simulink model "wrench_observer_R2016b"  (R2016b)
settings: Solver=VariableStepAuto  StartTime=0.0  StopTime=0.75  RelTol=1e-3
InitFcn:
  | %x_k1 = 0.00001*ones(36,1); % initialisation with initial state uncertainity
  | %P_k1 = 0.00001*ones(36); % initialisation with initial state uncertainity
values from neighbouring files (symbols this model uses):
  a_noise = 0    [parameter.m]
  alpha1 = pi/2    (= 1.57079632679)    [parameter.m]
  alpha2 = 0    [parameter.m]
  alpha3 = 0    [parameter.m]
  angular_noise = 0    [parameter.m]
  g = 9.81    [parameter.m]
  K_f_comm = 1    [parameter.m]
  K_I = [500*eye(3), zeros(3), zeros(3) ... (first row only)    [parameter.m]
  K_tau_comm = 1    [parameter.m]
  K_tau_man_comm = 1    [parameter.m]
  m = 3.9    [parameter.m]
  m_l1 = 0.3    [parameter.m]
  m_l2 = 0.35    [parameter.m]
  m_l3 = 0.35    [parameter.m]
  N_m = 1*diag([(p_noise/(3*noise_factor))^2 (p_noise/(3*noise_factor))^2 (p_noise/(3*noise_factor))^2 (a_noise/(3*noise_factor))^2 (a_noise/(3*noise_factor))^2 (a_noise/(3*noise_factor))^2 (angular_noise/(3*noise_factor))^2 (angular_noise/(3*noise_factor))^2 (angular_noise/(3*noise_factor))^2 (omega_noise/(3*noise_factor))^2 (omega_noise/(3*noise_factor))^2 (omega_noise/(3*noise_factor))^2 (theta_noise/( ...(+272 chars)    [parameter.m]
  N_p = diag(noise_factor_EKF)    [parameter.m]
  omega_dot_noise = 0    [parameter.m]
  omega_noise = 0    [parameter.m]
  p_L1_l1 = [p_L1_x_l1 p_L1_y_l1 p_L1_z_l1]'    [parameter.m]
  p_L2_l2 = [p_L2_x_l2 p_L2_y_l2 p_L2_z_l2]'    [parameter.m]
  p_L3_l3 = [p_L3_x_l3 p_L3_y_l3 p_L3_z_l3]'    [parameter.m]
  p_noise = 0    [parameter.m]
  R_B_L0 = [1 0 0;0 1 0; 0 0 1]    [parameter.m]
  T_delay = 0    [parameter.m]
  T_dis = 0.01    [parameter.m]
  theta_dot_dot_noise = 0    [parameter.m]
  theta_dot_noise = 0    [parameter.m]
  theta_noise = 0    [parameter.m]
  Ts = 1/250    (= 0.004)    [parameter.m]
  v_noise = 0    [parameter.m]
libraries: simulink x9, dspstat3 x2, dspinverses x1
(part 3 of 5)

== matlab function wrench_observer_R2016b/Wrench Observer EKF/MATLAB Function1 ==
  data: T_dis input; F output
function F = fcn(T_dis)
F = [ 	1, 	0, 	0, 	T_dis, 	0, 	0, 	0, 	0, 	0, 	0, 	0, 	0, 	0, 	0, 	0, 	0, 	0, 	0, 	0, 	0, 	0, 	0, 	0, 	0, 	0, 	0, 	0, 	0, 	0, 	0, 	0, 	0, 	0, 	0, 	0, 	0; 
		0, 	1, 	0, 	0, 	T_dis, 	0, 	0, 	0, 	0, 	0, 	0, 	0, 	0, 	0, 	0, 	0, 	0, 	0, 	0, 	0, 	0, 	0, 	0, 	0, 	0, 	0, 	0, 	0, 	0, 	0, 	0, 	0, 	0, 	0, 	0, 	0; 
		0, 	0, 	1, 	0, 	0, 	T_dis, 	0, 	0, 	0, 	0, 	0, 	0, 	0, 	0, 	0, 	0, 	0, 	0, 	0, 	0, 	0, 	0, 	0, 	0, 	0, 	0, 	0, 	0, 	0, 	0, 	0, 	0, 	0, 	0, 	0, 	0; 
		0, 	0, 	0, 	1, 	0, 	0, 	-(10*T_dis*((21*3^(1/2))/10000000000 + (3^(1/2)*((3*3^(1/2))/20 - 1/10))/2000000 - 3783/80000000000))/49, 	-(10*T_dis*((63*3^(1/2))/40000000000 + (3^(1/2)*((3*3^(1/2))/20 - 1/10))/2000000 + 52641/160000000000))/49, 	-(10*T_dis*((21*3^(1/2))/40000000000 + (3^(1/2)*((3*3^(1/2))/20 - 1/10))/1000000 + 53013/160000000000))/49, 	-(10*T_dis*((21*3^(1/2))/4000000 + 3/2000000))/49, 	(381*T_dis)/7840000, 	-(10*T_dis*((21*3^(1/2))/4000000 + (3^(1/2)*((3*3^(1/2))/20 - 1/10))/400 + 237/32000000))/49, 	(10*T_dis*((35937*3^(1/2))/1600000000000 + 1/100000000))/49, 	(10*T_dis*((35397*3^(1/2))/1600000000000 + 63/40000000000))/49, 	(10*T_dis*((177*3^(1/2))/80000000000 + 21/25000000000))/49, 	-(10*T_dis*((3*3^(1/2)*((3*3^(1/2))/20 - 1/10))/400 + 27/40000))/49, 	-(687*T_dis)/1600000, 	-(23643*T_dis)/156800000, 	(10*T_dis)/49, 	0, 	0, 	(10*T_dis)/49, 	0, 	0, 	0, 	0, 	0, 	0, 	0, 	0, 	0, 	0, 	0, 	0, 	0, 	0; 
		0, 	0, 	0, 	0, 	1, 	0, 	-(10*T_dis*((243969*3^(1/2))/800000000000 + 26389/50000000000))/49, 	(10*T_dis*((26073*3^(1/2))/400000000000 - 991/12500000000))/49, 	-(10*T_dis*((179727*3^(1/2))/800000000000 + 110003/200000000000))/49, 	-(381*T_dis)/784000, 	-(10*T_dis*((2121*3^(1/2))/80000000 + 303/40000000))/49, 	(10*T_dis*((56073*3^(1/2))/160000000 - 10303/40000000))/49, 	-(10*T_dis*((3^(1/2)*((3*3^(1/2))/20 - 1/10))/10000000 + 60189/1600000000000))/49, 	(10*T_dis*((249*3^(1/2))/80000000000 - 192873/1600000000000))/49, 	-(10*T_dis*((3561*3^(1/2))/160000000000 + 990219/8000000000000))/49, 	(10*T_dis*((3*3^(1/2))/8000 - 3/2000))/49, 	-(10*T_dis*((35979*3^(1/2))/16000000 + 3/2000))/49, 	-(10*T_dis*((23979*3^(1/2))/32000000 + 21/160000))/49, 	0, 	(10*T_dis)/49, 	0, 	0, 	(10*T_dis)/49, 	0, 	0, 	0, 	0, 	0, 	0, 	0, 	0, 	0, 	0, 	0, 	0, 	0; 
		0, 	0, 	0, 	0, 	0, 	1, 	(10*T_dis*((39969*3^(1/2))/80000000000 + (3^(1/2)*((3*3^(1/2))/20 - 1/10))/2000000 + 5337/40000000000))/49, 	(10*T_dis*((3^(1/2)*((3*3^(1/2))/20 - 1/10))/2000000 - (24273*3^(1/2))/80000000000 + 10003/20000000000))/49, 	(10*T_dis*((3927*3^(1/2))/80000000000 + 5331/40000000000))/49, 	(10*T_dis*((21*3^(1/2))/40000 + (3^(1/2)*((3*3^(1/2))/20 - 1/10))/400 + 237/320000))/49, 	-(10*T_dis*((60231*3^(1/2))/16000000 - 5003/2000000))/49, 	0, 	(10*T_dis*((183*3^(1/2))/16000000000 + (3^(1/2)*((3*3^(1/2))/20 - 1/10))/2000000 - 611/160000000000))/49, 	-(10*T_dis*((14871*3^(1/2))/800000000000 - 24147/160000000000))/49, 	-(10*T_dis*((24021*3^(1/2))/1600000000000 - 17601/200000000000))/49, 	(10*T_dis*((3^(1/2)*((3*3^(1/2))/20 - 1/10))/400 - (9*3^(1/2))/4000 + 1/400))/49, 	(10*T_dis*((2379*3^(1/2))/1600000 + 63/160000))/49, 	(10*T_dis*((4779*3^(1/2))/3200000 + 63/320000))/49, 	0, 	0, 	(10*T_dis)/49, 	0, 	0, 	(10*T_dis)/49, 	0, 	0, 	0, 	0, 	0, 	0, 	0, 	0, 	0, 	0, 	0, 	0; 
		0, 	0, 	0, 	0, 	0, 	0, 	(T_dis*(cos(1/10)/100000 - sin(1/10)/100000))/(cos(1/10)^2 + sin(1/10)^2) + 1, 	0, 	0, 	T_dis, 	(T_dis*sin(1/10))/(cos(1/10)^2 + sin(1/10)^2), 	(T_dis*cos(1/10))/(cos(1/10)^2 + sin(1/10)^2), 	0, 	0, 	0, 	0, 	0, 	0, 	0, 	0, 	0, 	0, 	0, 	0, 	0, 	0, 	0, 	0, 	0, 	0, 	0, 	0, 	0, 	0, 	0, 	0; 
		0, 	0, 	0, 	0, 	0, 	0, 	-(T_dis*(cos(1/10)/100000 + sin(1/10)/100000))/(cos(1/10)^2 + sin(1/10)^2), 	1, 	0, 	0, 	(T_dis*cos(1/10))/(cos(1/10)^2 + sin(1/10)^2), 	-(T_dis*sin(1/10))/(cos(1/10)^2 + sin(1/10)^2), 	0, 	0, 	0, 	0, 	0, 	0, 	0, 	0, 	0, 	0, 	0, 	0, 	0, 	0, 	0, 	0, 	0, 	0, 	0, 	0, 	0, 	0, 	0, 	0; 
		0, 	0, 	0, 	0, 	0, 	0, 	(T_dis*(cos(1/10)/100000 - sin(1/10)/100000))/(cos(1/10)*(cos(1/10)^2 + sin(1/10)^2)), 	(T_dis*sin(1/10)*(cos(1/10)/100000 + sin(1/10)/100000))/(cos(1/10)^2*(cos(1/10)^2 + sin(1/10)^2)), 	1, 	0, 	(T_dis*sin(1/10))/(cos(1/10)*(cos(1/10)^2 + sin(1/10)^2)), 	T_dis/(cos(1/10)^2 + sin(1/10)^2), 	0, 	0, 	0, 	0, 	0, 	0, 	0, 	0, 	0, 	0, 	0, 	0, 	0, 	0, 	0, 	0, 	0, 	0, 	0, 	0, 	0, 	0, 	0, 	0; 
		0, 	0, 	0, 	-T_dis*((5678455*3^(1/2))/877074 - 11415/292358), 	T_dis*((41050000000*3^(1/2)*((2121*3^(1/2))/80000000 + 303/40000000))/1315611 + 32247375/584716), 	T_dis*((41050000000*3^(1/2)*((11937*3^(1/2))/3200000 - 1/400))/1315611 - (9512500*3^(1/2)*((3*3^(1/2))/20 - 1/10))/146179 + 17978625/1169432), 	-T_dis*((41050000000*3^(1/2)*((3185121*3^(1/2))/1600000000000000 + 28784631/800000000000000))/1315611 - (20898335275230313*3^(1/2))/32821708862976000000 + (124478660218750000*3^(1/2)*((1196771067*3^(1/2))/16000000000000000 + 638273444637/32000000000000000))/192314700369 + (24547528595*3^(1/2)*((3*3^(1/2))/20 - 1/10))/4102713607872 + 268511624179821543629/656434177259520000000), 	-T_dis*((63720582757786447*3^(1/2))/98465126588928000000 - (41050000000*3^(1/2)*((1199798391*3^(1/2))/1600000000000000 - 3443358149/6400000000000000))/1315611 + (192991315468750000*3^(1/2)*((1196771067*3^(1/2))/16000000000000000 + 638273444637/32000000000000000))/576944101107 - (79106538965*3^(1/2)*((3*3^(1/2))/20 - 1/10))/12308140823616 + 20428475245687929968893/1969302531778560000000), 	-T_dis*((41050000000*3^(1/2)*((12396063*3^(1/2))/3200000000000000 + 59490177/1280000000000000))/1315611 + (31780980385867259*3^(1/2))/24616281647232000000 + (333669896375000000*3^(1/2)*((1196771067*3^(1/2))/16000000000000000 + 638273444637/32000000000000000))/576944101107 - (38681210545*3^(1/2)*((3*3^(1/2))/20 - 1/10))/3077035205904 + 4954579914681820686731/492325632944640000000), 	1 - (1927715899*3^(1/2)*T_dis)/5613273600, 	(1655290277*T_dis)/18710912000, 	T_dis*((17996889*3^(1/2))/467772800 + (41050000000*3^(1/2)*((16870959*3^(1/2))/640000000000 + 2152887/640000000000))/1315611 + 2040702927/18710912000), 	-T_dis*((278322450041*3^(1/2))/58471600000000 + (41050000000*3^(1/2)*((3^(1/2)*((3*3^(1/2))/20 - 1/10))/4000000 - (395710537*3^(1/2))/16000000000000000 + 3530354301/32000000000000000))/1315611 + (8210000000*3^(1/2)*((3935023*3^(1/2))/1600000000000000 - (3^(1/2)*((3*3^(1/2))/20 - 1/10))/40000000 + 641376324757/32000000000000000))/1315611 + 174654816435461/140331840000000), 	-T_dis*((41050000000*3^(1/2)*((108595719*3^(1/2))/4000000000000000 + 352356880263/1600000000000000000))/1315611 - (98168671543069*3^(1/2))/50659312000000000 + (2800*3^(1/2)*((3*3^(1/2))/20 - 1/10))/3166207 + 34794801151665391/49139532640000000), 	-T_dis*((41050000000*3^(1/2)*((498635583*3^(1/2))/32000000000000000 + 473633833263/3200000000000000000))/1315611 - (1241225136693592573*3^(1/2))/673211597168000000000 - (280000000*3^(1/2)*((3935023*3^(1/2))/1600000000000000 - (3^(1/2)*((3*3^(1/2))/20 - 1/10))/40000000 + 641376324757/32000000000000000))/2271049 + (1400*3^(1/2)*((3*3^(1/2))/20 - 1/10))/3166207 + 1886791839563181847/6732115971680000000), 	T_dis*((3000470039*3^(1/2))/467772800 + (41050000000*3^(1/2)*((23855781*3^(1/2))/6400000000 - 409671889/160000000000))/1315611 - 9176835837/935545600), 	T_dis*((20547*3^(1/2))/2338864 - (41050000000*3^(1/2)*((7774851*3^(1/2))/320000000000 + 114087/800000000))/1315611 + 46112862729/935545600), 	T_dis*((93603*3^(1/2))/37421824 - (41050000000*3^(1/2)*((2116647*3^(1/2))/320000000000 - 168129/12800000000))/1315611 + 1609129173/935545600), 	0, 	0, 	0, 	0, 	0, 	0, 	(3805000000*T_dis)/146179, 	(41050000000*3^(1/2)*T_dis)/1315611, 	0, 	(3805000000*T_dis)/146179, 	(41050000000*3^(1/2)*T_dis)/1315611, 	0, 	0, 	0, 	0, 	0, 	0, 	0; 
		0, 	0, 	0, 	T_dis*((41050000000*3^(1/2)*((21*3^(1/2))/4000000 + 3/2000000))/1315611 - 599676875/877074), 	T_dis*((266044675*3^(1/2))/1754148 + 21439775/877074), 	-T_dis*((41050000000*3^(1/2)*((3^(1/2)*((3*3^(1/2))/20 - 1/10))/400 - 189/320000))/1315611 - (21116055625*3^(1/2))/1754148 + 10613750000/1315611), 	-T_dis*((31682374967949716401*3^(1/2))/3282170886297600000 - (41050000000*3^(1/2)*((1057699*3^(1/2))/40000000000000 - (3^(1/2)*((3*3^(1/2))/20 - 1/10))/4000000 + 43060533/100000000000000))/1315611 + (124478660218750000*3^(1/2)*((3935023*3^(1/2))/1600000000000000 - (3^(1/2)*((3*3^(1/2))/20 - 1/10))/40000000 + 641376324757/32000000000000000))/192314700369 + 3377333141168213713051/1312868354519040000), 	-T_dis*((41050000000*3^(1/2)*((3^(1/2)*((3*3^(1/2))/20 - 1/10))/4000000 - (384367*3^(1/2))/16000000000000 + 173118651/1280000000000000))/1315611 - (2417983914522761711*3^(1/2))/1094056962099200000 + (192991315468750000*3^(1/2)*((3935023*3^(1/2))/1600000000000000 - (3^(1/2)*((3*3^(1/2))/20 - 1/10))/40000000 + 641376324757/32000000000000000))/576944101107 + 1135673785451784445223/19693025317785600000), 	-T_dis*((41050000000*3^(1/2)*((167139*3^(1/2))/80000000000000 - 3627028521/6400000000000000))/1315611 + (761268271444859597*3^(1/2))/164108544314880000 + (333669896375000000*3^(1/2)*((3935023*3^(1/2))/1600000000000000 - (3^(1/2)*((3*3^(1/2))/20 - 1/10))/40000000 + 641376324757/32000000000000000))/576944101107 + 6074430343735897953581/4923256329446400000), 	-(8782192229*T_dis)/561327360, 	(1966826299*3^(1/2)*T_dis)/5613273600 + 1, 	T_dis*((15916812541*3^(1/2))/187109120 + (41050000000*3^(1/2)*((23649*3^(1/2))/16000000000 + 2681607/640000000000))/1315611 + 553944349/51029760), 	-T_dis*((235405*3^(1/2)*((3*3^(1/2))/20 - 1/10))/292358 - (821000000000*3^(1/2)*((1196771067*3^(1/2))/16000000000000000 + 638273444637/32000000000000000))/1315611 - (1117838953967*3^(1/2))/14033184000000 + (41050000000*3^(1/2)*((14171247*3^(1/2))/4000000000000000 - 4237753/800000000000000))/1315611 + 169112788618613/105248880000000), 	-T_dis*((102454027781*3^(1/2))/1169432000000 + (1120000000000*3^(1/2)*((3^(1/2)*((3*3^(1/2))/20 - 1/10))/40000000 - (1688882473*3^(1/2))/160000000000000000 + 640513622513/32000000000000000))/3166207 - (41050000000*3^(1/2)*((4808147313*3^(1/2))/80000000000000000 - 1314171/800000000000000))/1315611 + 997287423437711/1403318400000000), 	-T_dis*((2126451751199909*3^(1/2))/42296016576000000 - (41050000000*3^(1/2)*((4242488889*3^(1/2))/80000000000000000 - 140757/160000000000000))/1315611 - (84000000000*3^(1/2)*((1196771067*3^(1/2))/16000000000000000 + 638273444637/32000000000000000))/2271049 + (560000000000*3^(1/2)*((3^(1/2)*((3*3^(1/2))/20 - 1/10))/40000000 - (1688882473*3^(1/2))/160000000000000000 + 640513622513/32000000000000000))/3166207 + (210*3^(1/2)*((3*3^(1/2))/20 - 1/10))/2271049 + 1706640172853415317/4229601657600000000), 	T_dis*((41050000000*3^(1/2)*((3942799*3^(1/2))/16000000000 - 12058917/32000000000))/1315611 + (337599060785*3^(1/2))/28066368 - 316229455409/38272320), 	-T_dis*((22005419947*3^(1/2))/280663680 - (41050000000*3^(1/2)*((27*3^(1/2))/80000000 + 60595089/32000000000))/1315611 + 1614521195/3508296), 	T_dis*((41050000000*3^(1/2)*((123*3^(1/2))/1280000000 + 2114493/32000000000))/1315611 - (1996938853*3^(1/2))/93554560 + 793101855/18710912), 	0, 	0, 	0, 	0, 	0, 	0, 	(41050000000*3^(1/2)*T_dis)/1315611, 	(4245500000000*T_dis)/1315611, 	0, 	(41050000000*3^(1/2)*T_dis)/1315611, 	(4245500000000*T_dis)/1315611, 	0, 	0, 	0, 	0, 	0, 	0, 	0; 
		0, 	0, 	0, 	-T_dis*((2800000*3^(1/2))/2101 - (4000000000*3^(1/2)*((3*3^(1/2))/20 - 1/10))/6303 + 3950000/2101), 	-T_dis*((213090000*3^(1/2))/2101 - 387880000/6303), 	0, 	-T_dis*((839000000*3^(1/2)*((3*3^(1/2))/20 - 1/10))/4414201 - (2185376953257*3^(1/2))/22071005000 + 10750848923274763/52970412000), 	-T_dis*((3349000000*3^(1/2)*((3*3^(1/2))/20 - 1/10))/13242603 - (5625435198179*3^(1/2))/66213015000 + 5362373015581261/26485206000), 	-T_dis*((653958112367*3^(1/2))/26485206000 - (823600000*3^(1/2)*((3*3^(1/2))/20 - 1/10))/13242603 + 51615522096961/52970412000), 	-T_dis*((747250*3^(1/2))/2101 - 3799095/4202), 	-T_dis*((28200995*3^(1/2))/4202 + 3572595/4202), 	1 - (21*3^(1/2)*T_dis)/4202, 	T_dis*((19901801*3^(1/2))/15757500 + (40000*3^(1/2)*((3*3^(1/2))/20 - 1/10))/6303 + 194049803/126060000), 	-T_dis*((2022620565609*3^(1/2))/316620700000 + (1120000000000*3^(1/2)*((1196771067*3^(1/2))/16000000000000000 + 638273444637/32000000000000000))/3166207 - (2800*3^(1/2)*((3*3^(1/2))/20 - 1/10))/3166207 - 28993407669249/6332414000000), 	-T_dis*((2622866155399*3^(1/2))/633241400000 + (560000000000*3^(1/2)*((1196771067*3^(1/2))/16000000000000000 + 638273444637/32000000000000000))/3166207 + (11200000000000*3^(1/2)*((3^(1/2)*((3*3^(1/2))/20 - 1/10))/40000000 - (1688882473*3^(1/2))/160000000000000000 + 640513622513/32000000000000000))/4414201 - (1400*3^(1/2)*((3*3^(1/2))/20 - 1/10))/3166207 - 42011537894569/12664828000000), 	-T_dis*((999902575*3^(1/2))/6303 - 2200952740/6303), 	T_dis*((713875*3^(1/2))/2101 - 2060250/2101), 	T_dis*((363917*3^(1/2))/2101 - 1009725/2101), 	0, 	0, 	0, 	0, 	0, 	0, 	0, 	0, 	(1600000000000*T_dis)/6303, 	0, 	0, 	(1600000000000*T_dis)/6303, 	0, 	0, 	0, 	0, 	0, 	0; 
		0, 	0, 	0, 	0, 	0, 	0, 	0, 	0, 	0, 	0, 	0, 	0, 	1, 	0, 	0, 	T_dis, 	0, 	0, 	0, 	0, 	0, 	0, 	0, 	0, 	0, 	0, 	0, 	0, 	0, 	0, 	0, 	0, 	0, 	0, 	0, 	0; 
		0, 	0, 	0, 	0, 	0, 	0, 	0, 	0, 	0, 	0, 	0, 	0, 	0, 	1, 	0, 	0, 	T_dis, 	0, 	0, 	0, 	0, 	0, 	0, 	0, 	0, 	0, 	0, 	0, 	0, 	0, 	0, 	0, 	0, 	0, 	0, 	0; 
		0, 	0, 	0, 	0, 	0, 	0, 	0, 	0, 	0, 	0, 	0, 	0, 	0, 	0, 	1, 	0, 	0, 	T_dis, 	0, 	0, 	0, 	0, 	0, 	0, 	0, 	0, 	0, 	0, 	0, 	0, 	0, 	0, 	0, 	0, 	0, 	0; 
		0, 	0, 	0, 	T_dis*(((3^(1/2)*((3*3^(1/2))/20 - 1/10))/400 + 27/40000)/(100*((3*3^(1/2))/100000000 - 31/400000000)) + 28569/(6400000000*((3*3^(1/2))/100000000 - 31/400000000))), 	T_dis*(((3*3^(1/2))/8000 + 1/1000)/(100*((3*3^(1/2))/100000000 - 31/400000000)) - ((21*3^(1/2))/16000000 + 3/2000)/(200*((3*3^(1/2))/100000000 - 31/400000000)) + ((23979*3^(1/2))/32000000 + 21/160000)/(200*((3*3^(1/2))/100000000 - 31/400000000))), 	-T_dis*(((4779*3^(1/2))/3200000 + 63/320000)/(200*((3*3^(1/2))/100000000 - 31/400000000)) - ((21*3^(1/2))/1600000 - 63/160000)/(200*((3*3^(1/2))/100000000 - 31/400000000)) + ((3^(1/2)*((3*3^(1/2))/20 - 1/10))/400 - (9*3^(1/2))/4000 + 1/400)/(100*((3*3^(1/2))/100000000 - 31/400000000))), 	T_dis*(((5121*3^(1/2)*((3*3^(1/2))/20 - 1/10))/40000000000000 - (4876773983*3^(1/2))/32000000000000000 + 111056949/800000000000000)/(100*((3*3^(1/2))/100000000 - 31/400000000)) - ((9397082859*3^(1/2))/64000000000000000 + (21*3^(1/2)*((3*3^(1/2))/20 - 1/10))/160000000000 + 346647/20000000000000)/(200*((3*3^(1/2))/100000000 - 31/400000000)) - ((1183480443*3^(1/2))/80000000000000000 + (21*3^(1/2)*((3*3^(1/2))/20 - 1/10))/3200000000000 - 16010785891/800000000000000)/(10*((3*3^(1/2))/100000000 - 31/400000000)) + ((1665944541*3^(1/2))/32000000000000000 + (3831*3^(1/2)*((3*3^(1/2))/20 - 1/10))/200000000000000 - 160128933757/8000000000000000)/(5*((3*3^(1/2))/100000000 - 31/400000000)) + ((377787*3^(1/2))/200000000000000 - 27893859/80000000000000)/(200*((3*3^(1/2))/100000000 - 31/400000000)) + ((5185251*3^(1/2))/16000000000000000 + 31944083711/1600000000000000)/(10*((3*3^(1/2))/100000000 - 31/400000000)) - (((21*3^(1/2))/20000000 - 217/80000000)*((5185251*3^(1/2))/16000000000000000 + 31944083711/1600000000000000))/(200*((3*3^(1/2))/100000000 - 31/400000000)^2) + (((21*3^(1/2))/20000000 - 217/80000000)*((1183480443*3^(1/2))/80000000000000000 + (21*3^(1/2)*((3*3^(1/2))/20 - 1/10))/3200000000000 - 16010785891/800000000000000))/(200*((3*3^(1/2))/100000000 - 31/400000000)^2) - (((21*3^(1/2))/20000000 - 217/80000000)*((1665944541*3^(1/2))/32000000000000000 + (3831*3^(1/2)*((3*3^(1/2))/20 - 1/10))/200000000000000 - 160128933757/8000000000000000))/(100*((3*3^(1/2))/100000000 - 31/400000000)^2)), 	-T_dis*(((1183480443*3^(1/2))/80000000000000000 + (21*3^(1/2)*((3*3^(1/2))/20 - 1/10))/3200000000000 - 16010785891/800000000000000)/(10*((3*3^(1/2))/100000000 - 31/400000000)) + ((3795389037*3^(1/2))/12800000000000000 + (21*3^(1/2)*((3*3^(1/2))/20 - 1/10))/320000000000 - 27840879/160000000000000)/(200*((3*3^(1/2))/100000000 - 31/400000000)) - ((1665944541*3^(1/2))/32000000000000000 + (3831*3^(1/2)*((3*3^(1/2))/20 - 1/10))/200000000000000 - 160128933757/8000000000000000)/(5*((3*3^(1/2))/100000000 - 31/400000000)) + ((2482807*3^(1/2)*((3*3^(1/2))/20 - 1/10))/5000000000000 - (11772968963*3^(1/2))/32000000000000000 + 61404471/200000000000000)/(100*((3*3^(1/2))/100000000 - 31/400000000)) - ((3210399*3^(1/2))/800000000000000 - (3*3^(1/2)*((3*3^(1/2))/20 - 1/10))/2000000000 + 4331121/160000000000000)/(200*((3*3^(1/2))/100000000 - 31/400000000)) - ((5185251*3^(1/2))/16000000000000000 + 31944083711/1600000000000000)/(10*((3*3^(1/2))/100000000 - 31/400000000)) - (((3*3^(1/2))/4000000 - 31/16000000)*((1183480443*3^(1/2))/80000000000000000 + (21*3^(1/2)*((3*3^(1/2))/20 - 1/10))/3200000000000 - 16010785891/800000000000000))/(200*((3*3^(1/2))/100000000 - 31/400000000)^2) + (((3*3^(1/2))/4000000 - 31/16000000)*((1665944541*3^(1/2))/32000000000000000 + (3831*3^(1/2)*((3*3^(1/2))/20 - 1/10))/200000000000000 - 160128933757/8000000000000000))/(100*((3*3^(1/2))/100000000 - 31/400000000)^2) + (((3*3^(1/2))/4000000 - 31/16000000)*((5185251*3^(1/2))/16000000000000000 + 31944083711/1600000000000000))/(200*((3*3^(1/2))/100000000 - 31/400000000)^2)), 	T_dis*(((114343521*3^(1/2))/1600000000000000 + (9943777*3^(1/2)*((3*3^(1/2))/20 - 1/10))/20000000000000 + 268316551/800000000000000)/(100*((3*3^(1/2))/100000000 - 31/400000000)) + ((3465639*3^(1/2))/1600000000000000 + (3*3^(1/2)*((3*3^(1/2))/20 - 1/10))/2000000000 - 55575441/160000000000000)/(200*((3*3^(1/2))/100000000 - 31/400000000)) + ((2404758213*3^(1/2))/16000000000000000 - (21*3^(1/2)*((3*3^(1/2))/20 - 1/10))/320000000000 + 7131903/64000000000000)/(200*((3*3^(1/2))/100000000 - 31/400000000)) + (((3*3^(1/2))/5000000 - 31/20000000)*((1183480443*3^(1/2))/80000000000000000 + (21*3^(1/2)*((3*3^(1/2))/20 - 1/10))/3200000000000 - 16010785891/800000000000000))/(200*((3*3^(1/2))/100000000 - 31/400000000)^2) - (((3*3^(1/2))/5000000 - 31/20000000)*((1665944541*3^(1/2))/32000000000000000 + (3831*3^(1/2)*((3*3^(1/2))/20 - 1/10))/200000000000000 - 160128933757/8000000000000000))/(100*((3*3^(1/2))/100000000 - 31/400000000)^2) - (((3*3^(1/2))/5000000 - 31/20000000)*((5185251*3^(1/2))/16000000000000000 + 31944083711/1600000000000000))/(200*((3*3^(1/2))/100000000 - 31/400000000)^2)), 	-T_dis*(((62493*3^(1/2))/16000000000 + (249937*3^(1/2)*((3*3^(1/2))/20 - 1/10))/100000000 - 23974611/32000000000)/(100*((3*3^(1/2))/100000000 - 31/400000000)) + 60604689/(6400000000000*((3*3^(1/2))/100000000 - 31/400000000)) + ((207*3^(1/2))/1280000000 + (21*3^(1/2)*((3*3^(1/2))/20 - 1/10))/32000000 + 2114643/32000000000)/(200*((3*3^(1/2))/100000000 - 31/400000000))), 	T_dis*(((2107047*3^(1/2))/320000000000 - 168129/12800000000)/(200*((3*3^(1/2))/100000000 - 31/400000000)) + ((7765251*3^(1/2))/320000000000 + 5703/40000000)/(200*((3*3^(1/2))/100000000 - 31/400000000)) - ((3*3^(1/2)*((3*3^(1/2))/20 - 1/10))/8000000000 - (596441019*3^(1/2))/160000000000 + 204842381/80000000000)/(100*((3*3^(1/2))/100000000 - 31/400000000))), 	-T_dis*(((416349*3^(1/2))/320000000000 - 123711/32000000000)/(200*((3*3^(1/2))/100000000 - 31/400000000)) + ((1031871*3^(1/2))/1600000000000 - 121359/64000000000)/(200*((3*3^(1/2))/100000000 - 31/400000000)) - ((20010287*3^(1/2)*((3*3^(1/2))/20 - 1/10))/8000000000 - (119986137*3^(1/2))/320000000000 + 40005943/160000000000)/(100*((3*3^(1/2))/100000000 - 31/400000000))), 	-T_dis*(((4034511*3^(1/2))/1600000000000000 + (297*3^(1/2)*((3*3^(1/2))/20 - 1/10))/400000000000 + 16684749/16000000000000000)/(200*((3*3^(1/2))/100000000 - 31/400000000)) + ((7589019*3^(1/2))/500000000000000 + (179409213*3^(1/2)*((3*3^(1/2))/20 - 1/10))/400000000000000 - 125998557/8000000000000000)/(100*((3*3^(1/2))/100000000 - 31/400000000)) + ((52161039*3^(1/2))/3200000000000000 + (21*3^(1/2)*((3*3^(1/2))/20 - 1/10))/32000000000000 - 117174411/8000000000000000)/(200*((3*3^(1/2))/100000000 - 31/400000000))), 	T_dis*(((1183480443*3^(1/2))/80000000000000000 + (21*3^(1/2)*((3*3^(1/2))/20 - 1/10))/3200000000000 - 16010785891/800000000000000)/(300*((3*3^(1/2))/100000000 - 31/400000000)) + ((78898791*3^(1/2))/4000000000000000 + (21*3^(1/2)*((3*3^(1/2))/20 - 1/10))/16000000000000 + 2373464247/20000000000000000)/(200*((3*3^(1/2))/100000000 - 31/400000000)) + ((29906877*3^(1/2))/1600000000000000 + (21*3^(1/2)*((3*3^(1/2))/20 - 1/10))/32000000000000 + 5990219349/80000000000000000)/(200*((3*3^(1/2))/100000000 - 31/400000000)) + ((5185251*3^(1/2))/16000000000000000 + 31944083711/1600000000000000)/(300*((3*3^(1/2))/100000000 - 31/400000000)) - ((23697*3^(1/2)*((3*3^(1/2))/20 - 1/10))/32000000000000 - (369986349*3^(1/2))/8000000000000000 + 51614439/8000000000000000)/(100*((3*3^(1/2))/100000000 - 31/400000000))), 	T_dis*(((599887743*3^(1/2))/16000000000000000 - (1779879*3^(1/2)*((3*3^(1/2))/20 - 1/10))/1600000000000000 + 14540151/32000000000000000)/(100*((3*3^(1/2))/100000000 - 31/400000000)) + ((11901*3^(1/2)*((3*3^(1/2))/20 - 1/10))/32000000000000 - (4750881*3^(1/2))/2000000000000000 + 4731132549/80000000000000000)/(200*((3*3^(1/2))/100000000 - 31/400000000)) + ((29900577*3^(1/2))/1600000000000000 + (21*3^(1/2)*((3*3^(1/2))/20 - 1/10))/32000000000000 + 5997450849/80000000000000000)/(200*((3*3^(1/2))/100000000 - 31/400000000)) + (((11*3^(1/2))/200000000 - 3/40000000)*((5185251*3^(1/2))/16000000000000000 + 31944083711/1600000000000000))/(200*((3*3^(1/2))/100000000 - 31/400000000)^2) - (100*((3*3^(1/2))/20000 - 1/20000)*((1183480443*3^(1/2))/80000000000000000 + (21*3^(1/2)*((3*3^(1/2))/20 - 1/10))/3200000000000 - 16010785891/800000000000000))/(3*((3*3^(1/2))/100000000 - 31/400000000)) - (((11*3^(1/2))/200000000 - 3/40000000)*((1183480443*3^(1/2))/80000000000000000 + (21*3^(1/2)*((3*3^(1/2))/20 - 1/10))/3200000000000 - 16010785891/800000000000000))/(200*((3*3^(1/2))/100000000 - 31/400000000)^2) + (((11*3^(1/2))/200000000 - 3/40000000)*((1665944541*3^(1/2))/32000000000000000 + (3831*3^(1/2)*((3*3^(1/2))/20 - 1/10))/200000000000000 - 160128933757/8000000000000000))/(100*((3*3^(1/2))/100000000 - 31/400000000)^2) + (3^(1/2)*((1665944541*3^(1/2))/32000000000000000 + (3831*3^(1/2)*((3*3^(1/2))/20 - 1/10))/200000000000000 - 160128933757/8000000000000000))/(100*((3*3^(1/2))/100000000 - 31/400000000)) + (100*((3*3^(1/2))/20000 + 1/20000)*((5185251*3^(1/2))/16000000000000000 + 31944083711/1600000000000000))/(3*((3*3^(1/2))/100000000 - 31/400000000))), 	1 - T_dis*(((891*3^(1/2))/80000000 - 417/40000000)/(100*((3*3^(1/2))/100000000 - 31/400000000)) + ((1192731*3^(1/2))/3200000000 - 1205067/3200000000)/(200*((3*3^(1/2))/100000000 - 31/400000000)) + ((292941*3^(1/2))/800000000 - 589209/1600000000)/(200*((3*3^(1/2))/100000000 - 31/400000000))), 	-T_dis*((9*3^(1/2))/(400000000*((3*3^(1/2))/100000000 - 31/400000000)) + ((58929*3^(1/2))/160000000 - 601209/1600000000)/(200*((3*3^(1/2))/100000000 - 31/400000000)) + ((307161*3^(1/2))/800000000 - 620169/1600000000)/(100*((3*3^(1/2))/100000000 - 31/400000000))), 	T_dis*(((58929*3^(1/2))/160000000 - 601209/1600000000)/(200*((3*3^(1/2))/100000000 - 31/400000000)) - ((1192731*3^(1/2))/3200000000 - 1205067/3200000000)/(100*((3*3^(1/2))/100000000 - 31/400000000))), 	0, 	0, 	0, 	0, 	0, 	0, 	0, 	0, 	0, 	0, 	0, 	0, 	-T_dis/(100*((3*3^(1/2))/100000000 - 31/400000000)), 	T_dis/(200*((3*3^(1/2))/100000000 - 31/400000000)), 	T_dis/(200*((3*3^(1/2))/100000000 - 31/400000000)), 	-T_dis/(100*((3*3^(1/2))/100000000 - 31/400000000)), 	T_dis/(200*((3*3^(1/2))/100000000 - 31/400000000)), 	T_dis/(200*((3*3^(1/2))/100000000 - 31/400000000)); 
		0, 	0, 	0, 	-T_dis*((2627*((3*3^(1/2))/10000 - 11/20000))/(320000*((3*3^(1/2))/100000000 - 31/400000000)) - (821*((3*3^(1/2))/10000 - 1/1000))/(480000*((3*3^(1/2))/100000000 - 31/400000000)) + ((3^(1/2)*((3*3^(1/2))/20 - 1/10))/400 + 27/40000)/(200*((3*3^(1/2))/100000000 - 31/400000000))), 	-T_dis*(((3*3^(1/2))/8000 + 1/1000)/(200*((3*3^(1/2))/100000000 - 31/400000000)) + (100*((3*3^(1/2))/10000 - 1/1000)*((21*3^(1/2))/16000000 + 3/2000))/(9*((3*3^(1/2))/100000000 - 31/400000000)) + (100*((3*3^(1/2))/10000 - 11/20000)*((23979*3^(1/2))/32000000 + 21/160000))/(9*((3*3^(1/2))/100000000 - 31/400000000))), 	T_dis*(((3^(1/2)*((3*3^(1/2))/20 - 1/10))/400 - (9*3^(1/2))/4000 + 1/400)/(200*((3*3^(1/2))/100000000 - 31/400000000)) + (100*((3*3^(1/2))/10000 - 1/1000)*((21*3^(1/2))/1600000 - 63/160000))/(9*((3*3^(1/2))/100000000 - 31/400000000)) + (100*((3*3^(1/2))/10000 - 11/20000)*((4779*3^(1/2))/3200000 + 63/320000))/(9*((3*3^(1/2))/100000000 - 31/400000000))), 	T_dis*((100*((9*3^(1/2))/2000 - 57/8000)*((1183480443*3^(1/2))/80000000000000000 + (21*3^(1/2)*((3*3^(1/2))/20 - 1/10))/3200000000000 - 16010785891/800000000000000))/(9*((3*3^(1/2))/100000000 - 31/400000000)) - ((1665944541*3^(1/2))/32000000000000000 + (3831*3^(1/2)*((3*3^(1/2))/20 - 1/10))/200000000000000 - 160128933757/8000000000000000)/(10*((3*3^(1/2))/100000000 - 31/400000000)) - ((5121*3^(1/2)*((3*3^(1/2))/20 - 1/10))/40000000000000 - (4876773983*3^(1/2))/32000000000000000 + 111056949/800000000000000)/(200*((3*3^(1/2))/100000000 - 31/400000000)) + (100*((3*3^(1/2))/10000 - 11/20000)*((9397082859*3^(1/2))/64000000000000000 + (21*3^(1/2)*((3*3^(1/2))/20 - 1/10))/160000000000 + 346647/20000000000000))/(9*((3*3^(1/2))/100000000 - 31/400000000)) + (((21*3^(1/2))/20000000 - 217/80000000)*((1665944541*3^(1/2))/32000000000000000 + (3831*3^(1/2)*((3*3^(1/2))/20 - 1/10))/200000000000000 - 160128933757/8000000000000000))/(200*((3*3^(1/2))/100000000 - 31/400000000)^2) + (100*((3*3^(1/2))/10000 - 1/1000)*((377787*3^(1/2))/200000000000000 - 27893859/80000000000000))/(9*((3*3^(1/2))/100000000 - 31/400000000)) + (100*((9*3^(1/2))/2000 - 129/8000)*((5185251*3^(1/2))/16000000000000000 + 31944083711/1600000000000000))/(9*((3*3^(1/2))/100000000 - 31/400000000)) - (100*((3*3^(1/2))/10000 - 1/1000)*((21*3^(1/2))/20000000 - 217/80000000)*((5185251*3^(1/2))/16000000000000000 + 31944083711/1600000000000000))/(9*((3*3^(1/2))/100000000 - 31/400000000)^2) - (100*((3*3^(1/2))/10000 - 11/20000)*((21*3^(1/2))/20000000 - 217/80000000)*((1183480443*3^(1/2))/80000000000000000 + (21*3^(1/2)*((3*3^(1/2))/20 - 1/10))/3200000000000 - 16010785891/800000000000000))/(9*((3*3^(1/2))/100000000 - 31/400000000)^2)), 	T_dis*(((2482807*3^(1/2)*((3*3^(1/2))/20 - 1/10))/5000000000000 - (11772968963*3^(1/2))/32000000000000000 + 61404471/200000000000000)/(200*((3*3^(1/2))/100000000 - 31/400000000)) - ((1665944541*3^(1/2))/32000000000000000 + (3831*3^(1/2)*((3*3^(1/2))/20 - 1/10))/200000000000000 - 160128933757/8000000000000000)/(10*((3*3^(1/2))/100000000 - 31/400000000)) + (100*((3*3^(1/2))/2000 + 1/1600)*((1183480443*3^(1/2))/80000000000000000 + (21*3^(1/2)*((3*3^(1/2))/20 - 1/10))/3200000000000 - 16010785891/800000000000000))/(9*((3*3^(1/2))/100000000 - 31/400000000)) + (100*((3*3^(1/2))/10000 - 11/20000)*((3795389037*3^(1/2))/12800000000000000 + (21*3^(1/2)*((3*3^(1/2))/20 - 1/10))/320000000000 - 27840879/160000000000000))/(9*((3*3^(1/2))/100000000 - 31/400000000)) + (((3*3^(1/2))/4000000 - 31/16000000)*((1665944541*3^(1/2))/32000000000000000 + (3831*3^(1/2)*((3*3^(1/2))/20 - 1/10))/200000000000000 - 160128933757/8000000000000000))/(200*((3*3^(1/2))/100000000 - 31/400000000)^2) + (100*((3*3^(1/2))/10000 - 1/1000)*((3210399*3^(1/2))/800000000000000 - (3*3^(1/2)*((3*3^(1/2))/20 - 1/10))/2000000000 + 4331121/160000000000000))/(9*((3*3^(1/2))/100000000 - 31/400000000)) + (100*((3*3^(1/2))/2000 - 67/8000)*((5185251*3^(1/2))/16000000000000000 + 31944083711/1600000000000000))/(9*((3*3^(1/2))/100000000 - 31/400000000)) - (100*((3*3^(1/2))/10000 - 1/1000)*((3*3^(1/2))/4000000 - 31/16000000)*((5185251*3^(1/2))/16000000000000000 + 31944083711/1600000000000000))/(9*((3*3^(1/2))/100000000 - 31/400000000)^2) - (100*((3*3^(1/2))/10000 - 11/20000)*((3*3^(1/2))/4000000 - 31/16000000)*((1183480443*3^(1/2))/80000000000000000 + (21*3^(1/2)*((3*3^(1/2))/20 - 1/10))/3200000000000 - 16010785891/800000000000000))/(9*((3*3^(1/2))/100000000 - 31/400000000)^2)), 	-T_dis*(((114343521*3^(1/2))/1600000000000000 + (9943777*3^(1/2)*((3*3^(1/2))/20 - 1/10))/20000000000000 + 268316551/800000000000000)/(200*((3*3^(1/2))/100000000 - 31/400000000)) - (100*((3*3^(1/2))/500 - 31/2000)*((1183480443*3^(1/2))/80000000000000000 + (21*3^(1/2)*((3*3^(1/2))/20 - 1/10))/3200000000000 - 16010785891/800000000000000))/(9*((3*3^(1/2))/100000000 - 31/400000000)) - (100*((3*3^(1/2))/10000 - 1/1000)*((3465639*3^(1/2))/1600000000000000 + (3*3^(1/2)*((3*3^(1/2))/20 - 1/10))/2000000000 - 55575441/160000000000000))/(9*((3*3^(1/2))/100000000 - 31/400000000)) + (100*((3*3^(1/2))/10000 - 11/20000)*((2404758213*3^(1/2))/16000000000000000 - (21*3^(1/2)*((3*3^(1/2))/20 - 1/10))/320000000000 + 7131903/64000000000000))/(9*((3*3^(1/2))/100000000 - 31/400000000)) - (((3*3^(1/2))/5000000 - 31/20000000)*((1665944541*3^(1/2))/32000000000000000 + (3831*3^(1/2)*((3*3^(1/2))/20 - 1/10))/200000000000000 - 160128933757/8000000000000000))/(200*((3*3^(1/2))/100000000 - 31/400000000)^2) - (100*((3*3^(1/2))/500 - 31/2000)*((5185251*3^(1/2))/16000000000000000 + 31944083711/1600000000000000))/(9*((3*3^(1/2))/100000000 - 31/400000000)) + (100*((3*3^(1/2))/10000 - 1/1000)*((3*3^(1/2))/5000000 - 31/20000000)*((5185251*3^(1/2))/16000000000000000 + 31944083711/1600000000000000))/(9*((3*3^(1/2))/100000000 - 31/400000000)^2) + (100*((3*3^(1/2))/10000 - 11/20000)*((3*3^(1/2))/5000000 - 31/20000000)*((1183480443*3^(1/2))/80000000000000000 + (21*3^(1/2)*((3*3^(1/2))/20 - 1/10))/3200000000000 - 16010785891/800000000000000))/(9*((3*3^(1/2))/100000000 - 31/400000000)^2)), 	T_dis*(((62493*3^(1/2))/16000000000 + (249937*3^(1/2)*((3*3^(1/2))/20 - 1/10))/100000000 - 23974611/32000000000)/(200*((3*3^(1/2))/100000000 - 31/400000000)) - (20201563*((3*3^(1/2))/10000 - 1/1000))/(960000000*((3*3^(1/2))/100000000 - 31/400000000)) + (100*((3*3^(1/2))/10000 - 11/20000)*((207*3^(1/2))/1280000000 + (21*3^(1/2)*((3*3^(1/2))/20 - 1/10))/32000000 + 2114643/32000000000))/(9*((3*3^(1/2))/100000000 - 31/400000000))), 	T_dis*(((3*3^(1/2)*((3*3^(1/2))/20 - 1/10))/8000000000 - (596441019*3^(1/2))/160000000000 + 204842381/80000000000)/(200*((3*3^(1/2))/100000000 - 31/400000000)) - (100*((3*3^(1/2))/10000 - 11/20000)*((2107047*3^(1/2))/320000000000 - 168129/12800000000))/(9*((3*3^(1/2))/100000000 - 31/400000000)) + (100*((3*3^(1/2))/10000 - 1/1000)*((7765251*3^(1/2))/320000000000 + 5703/40000000))/(9*((3*3^(1/2))/100000000 - 31/400000000))), 	-T_dis*(((20010287*3^(1/2)*((3*3^(1/2))/20 - 1/10))/8000000000 - (119986137*3^(1/2))/320000000000 + 40005943/160000000000)/(200*((3*3^(1/2))/100000000 - 31/400000000)) + (100*((416349*3^(1/2))/320000000000 - 123711/32000000000)*((3*3^(1/2))/10000 - 1/1000))/(9*((3*3^(1/2))/100000000 - 31/400000000)) - (100*((3*3^(1/2))/10000 - 11/20000)*((1031871*3^(1/2))/1600000000000 - 121359/64000000000))/(9*((3*3^(1/2))/100000000 - 31/400000000))), 	T_dis*(((7589019*3^(1/2))/500000000000000 + (179409213*3^(1/2)*((3*3^(1/2))/20 - 1/10))/400000000000000 - 125998557/8000000000000000)/(200*((3*3^(1/2))/100000000 - 31/400000000)) - (100*((3*3^(1/2))/10000 - 1/1000)*((4034511*3^(1/2))/1600000000000000 + (297*3^(1/2)*((3*3^(1/2))/20 - 1/10))/400000000000 + 16684749/16000000000000000))/(9*((3*3^(1/2))/100000000 - 31/400000000)) + (100*((3*3^(1/2))/10000 - 11/20000)*((52161039*3^(1/2))/3200000000000000 + (21*3^(1/2)*((3*3^(1/2))/20 - 1/10))/32000000000000 - 117174411/8000000000000000))/(9*((3*3^(1/2))/100000000 - 31/400000000))), 	-T_dis*(((1665944541*3^(1/2))/32000000000000000 + (3831*3^(1/2)*((3*3^(1/2))/20 - 1/10))/200000000000000 - 160128933757/8000000000000000)/(300*((3*3^(1/2))/100000000 - 31/400000000)) + ((5185251*3^(1/2))/16000000000000000 + 31944083711/1600000000000000)/(300*((3*3^(1/2))/100000000 - 31/400000000)) - ((23697*3^(1/2)*((3*3^(1/2))/20 - 1/10))/32000000000000 - (369986349*3^(1/2))/8000000000000000 + 51614439/8000000000000000)/(200*((3*3^(1/2))/100000000 - 31/400000000)) - (100*((3*3^(1/2))/10000 - 1/1000)*((78898791*3^(1/2))/4000000000000000 + (21*3^(1/2)*((3*3^(1/2))/20 - 1/10))/16000000000000 + 2373464247/20000000000000000))/(9*((3*3^(1/2))/100000000 - 31/400000000)) + (100*((3*3^(1/2))/10000 - 11/20000)*((29906877*3^(1/2))/1600000000000000 + (21*3^(1/2)*((3*3^(1/2))/20 - 1/10))/32000000000000 + 5990219349/80000000000000000))/(9*((3*3^(1/2))/100000000 - 31/400000000))), 	-T_dis*(((599887743*3^(1/2))/16000000000000000 - (1779879*3^(1/2)*((3*3^(1/2))/20 - 1/10))/1600000000000000 + 14540151/32000000000000000)/(200*((3*3^(1/2))/100000000 - 31/400000000)) + ((5185251*3^(1/2))/16000000000000000 + 31944083711/1600000000000000)/(300*((3*3^(1/2))/100000000 - 31/400000000)) - (100*((9*3^(1/2))/20000 - 3/20000)*((1183480443*3^(1/2))/80000000000000000 + (21*3^(1/2)*((3*3^(1/2))/20 - 1/10))/3200000000000 - 16010785891/800000000000000))/(9*((3*3^(1/2))/100000000 - 31/400000000)) - (100*((3*3^(1/2))/10000 - 1/1000)*((11901*3^(1/2)*((3*3^(1/2))/20 - 1/10))/32000000000000 - (4750881*3^(1/2))/2000000000000000 + 4731132549/80000000000000000))/(9*((3*3^(1/2))/100000000 - 31/400000000)) + (100*((3*3^(1/2))/10000 - 11/20000)*((29900577*3^(1/2))/1600000000000000 + (21*3^(1/2)*((3*3^(1/2))/20 - 1/10))/32000000000000 + 5997450849/80000000000000000))/(9*((3*3^(1/2))/100000000 - 31/400000000)) + (100*((3*3^(1/2))/20000 + 1/20000)*((1665944541*3^(1/2))/32000000000000000 + (3831*3^(1/2)*((3*3^(1/2))/20 - 1/10))/200000000000000 - 160128933757/8000000000000000))/(3*((3*3^(1/2))/100000000 - 31/400000000)) + (((11*3^(1/2))/200000000 - 3/40000000)*((1665944541*3^(1/2))/32000000000000000 + (3831*3^(1/2)*((3*3^(1/2))/20 - 1/10))/200000000000000 - 160128933757/8000000000000000))/(200*((3*3^(1/2))/100000000 - 31/400000000)^2) - (100*((3*3^(1/2))/10000 - 1/1000)*((11*3^(1/2))/200000000 - 3/40000000)*((5185251*3^(1/2))/16000000000000000 + 31944083711/1600000000000000))/(9*((3*3^(1/2))/100000000 - 31/400000000)^2) - (100*((3*3^(1/2))/10000 - 11/20000)*((11*3^(1/2))/200000000 - 3/40000000)*((1183480443*3^(1/2))/80000000000000000 + (21*3^(1/2)*((3*3^(1/2))/20 - 1/10))/3200000000000 - 16010785891/800000000000000))/(9*((3*3^(1/2))/100000000 - 31/400000000)^2)), 	T_dis*(((891*3^(1/2))/80000000 - 417/40000000)/(200*((3*3^(1/2))/100000000 - 31/400000000)) + (100*((3*3^(1/2))/10000 - 11/20000)*((1192731*3^(1/2))/3200000000 - 1205067/3200000000))/(9*((3*3^(1/2))/100000000 - 31/400000000)) - (100*((3*3^(1/2))/10000 - 1/1000)*((292941*3^(1/2))/800000000 - 589209/1600000000))/(9*((3*3^(1/2))/100000000 - 31/400000000))), 	T_dis*(((307161*3^(1/2))/800000000 - 620169/1600000000)/(200*((3*3^(1/2))/100000000 - 31/400000000)) - (3^(1/2)*((3*3^(1/2))/10000 - 1/1000))/(20000*((3*3^(1/2))/100000000 - 31/400000000)) + (100*((3*3^(1/2))/10000 - 11/20000)*((58929*3^(1/2))/160000000 - 601209/1600000000))/(9*((3*3^(1/2))/100000000 - 31/400000000))) + 1, 	T_dis*(((1192731*3^(1/2))/3200000000 - 1205067/3200000000)/(200*((3*3^(1/2))/100000000 - 31/400000000)) + (100*((3*3^(1/2))/10000 - 1/1000)*((58929*3^(1/2))/160000000 - 601209/1600000000))/(9*((3*3^(1/2))/100000000 - 31/400000000))), 	0, 	0, 	0, 	0, 	0, 	0, 	0, 	0, 	0, 	0, 	0, 	0, 	T_dis/(200*((3*3^(1/2))/100000000 - 31/400000000)), 	(100*T_dis*((3*3^(1/2))/10000 - 1/1000))/(9*((3*3^(1/2))/100000000 - 31/400000000)), 	-(100*T_dis*((3*3^(1/2))/10000 - 11/20000))/(9*((3*3^(1/2))/100000000 - 31/400000000)), 	T_dis/(200*((3*3^(1/2))/100000000 - 31/400000000)), 	(100*T_dis*((3*3^(1/2))/10000 - 1/1000))/(9*((3*3^(1/2))/100000000 - 31/400000000)), 	-(100*T_dis*((3*3^(1/2))/10000 - 11/20000))/(9*((3*3^(1/2))/100000000 - 31/400000000)); 
		0, 	0, 	0, 	-T_dis*((821*((3*3^(1/2))/10000 - 11/20000))/(480000*((3*3^(1/2))/100000000 - 31/400000000)) + ((3^(1/2)*((3*3^(1/2))/20 - 1/10))/400 + 27/40000)/(200*((3*3^(1/2))/100000000 - 31/400000000)) - (2627*((27009*3^(1/2))/1000000000 - 3489/50000000))/(1600000*((9*3^(1/2))/50000000000000 - 93/200000000000000))), 	T_dis*((20*((23979*3^(1/2))/32000000 + 21/160000)*((27009*3^(1/2))/1000000000 - 3489/50000000))/(9*((9*3^(1/2))/50000000000000 - 93/200000000000000)) - ((3*3^(1/2))/8000 + 1/1000)/(200*((3*3^(1/2))/100000000 - 31/400000000)) + (100*((3*3^(1/2))/10000 - 11/20000)*((21*3^(1/2))/16000000 + 3/2000))/(9*((3*3^(1/2))/100000000 - 31/400000000))), 	-T_dis*((20*((4779*3^(1/2))/3200000 + 63/320000)*((27009*3^(1/2))/1000000000 - 3489/50000000))/(9*((9*3^(1/2))/50000000000000 - 93/200000000000000)) - ((3^(1/2)*((3*3^(1/2))/20 - 1/10))/400 - (9*3^(1/2))/4000 + 1/400)/(200*((3*3^(1/2))/100000000 - 31/400000000)) + (100*((3*3^(1/2))/10000 - 11/20000)*((21*3^(1/2))/1600000 - 63/160000))/(9*((3*3^(1/2))/100000000 - 31/400000000))), 	-T_dis*(((5121*3^(1/2)*((3*3^(1/2))/20 - 1/10))/40000000000000 - (4876773983*3^(1/2))/32000000000000000 + 111056949/800000000000000)/(200*((3*3^(1/2))/100000000 - 31/400000000)) + ((1665944541*3^(1/2))/32000000000000000 + (3831*3^(1/2)*((3*3^(1/2))/20 - 1/10))/200000000000000 - 160128933757/8000000000000000)/(10*((3*3^(1/2))/100000000 - 31/400000000)) + (20*((27009*3^(1/2))/1000000000 - 3489/50000000)*((9397082859*3^(1/2))/64000000000000000 + (21*3^(1/2)*((3*3^(1/2))/20 - 1/10))/160000000000 + 346647/20000000000000))/(9*((9*3^(1/2))/50000000000000 - 93/200000000000000)) - (((21*3^(1/2))/20000000 - 217/80000000)*((1665944541*3^(1/2))/32000000000000000 + (3831*3^(1/2)*((3*3^(1/2))/20 - 1/10))/200000000000000 - 160128933757/8000000000000000))/(200*((3*3^(1/2))/100000000 - 31/400000000)^2) + (100*((3*3^(1/2))/10000 - 11/20000)*((377787*3^(1/2))/200000000000000 - 27893859/80000000000000))/(9*((3*3^(1/2))/100000000 - 31/400000000)) + (20*((37809*3^(1/2))/40000000 - 1953627/800000000)*((1183480443*3^(1/2))/80000000000000000 + (21*3^(1/2)*((3*3^(1/2))/20 - 1/10))/3200000000000 - 16010785891/800000000000000))/(9*((9*3^(1/2))/50000000000000 - 93/200000000000000)) + (100*((9*3^(1/2))/2000 - 57/8000)*((5185251*3^(1/2))/16000000000000000 + 31944083711/1600000000000000))/(9*((3*3^(1/2))/100000000 - 31/400000000)) - (100*((3*3^(1/2))/10000 - 11/20000)*((21*3^(1/2))/20000000 - 217/80000000)*((5185251*3^(1/2))/16000000000000000 + 31944083711/1600000000000000))/(9*((3*3^(1/2))/100000000 - 31/400000000)^2) - (20*((27009*3^(1/2))/1000000000 - 3489/50000000)*((81*3^(1/2))/10000000000000 - 837/40000000000000)*((1183480443*3^(1/2))/80000000000000000 + (21*3^(1/2)*((3*3^(1/2))/20 - 1/10))/3200000000000 - 16010785891/800000000000000))/(9*((9*3^(1/2))/50000000000000 - 93/200000000000000)^2)), 	-T_dis*(((1665944541*3^(1/2))/32000000000000000 + (3831*3^(1/2)*((3*3^(1/2))/20 - 1/10))/200000000000000 - 160128933757/8000000000000000)/(10*((3*3^(1/2))/100000000 - 31/400000000)) - ((2482807*3^(1/2)*((3*3^(1/2))/20 - 1/10))/5000000000000 - (11772968963*3^(1/2))/32000000000000000 + 61404471/200000000000000)/(200*((3*3^(1/2))/100000000 - 31/400000000)) + (20*((27009*3^(1/2))/1000000000 - 3489/50000000)*((3795389037*3^(1/2))/12800000000000000 + (21*3^(1/2)*((3*3^(1/2))/20 - 1/10))/320000000000 - 27840879/160000000000000))/(9*((9*3^(1/2))/50000000000000 - 93/200000000000000)) - (((3*3^(1/2))/4000000 - 31/16000000)*((1665944541*3^(1/2))/32000000000000000 + (3831*3^(1/2)*((3*3^(1/2))/20 - 1/10))/200000000000000 - 160128933757/8000000000000000))/(200*((3*3^(1/2))/100000000 - 31/400000000)^2) + (20*((135063*3^(1/2))/200000000 - 1395921/800000000)*((1183480443*3^(1/2))/80000000000000000 + (21*3^(1/2)*((3*3^(1/2))/20 - 1/10))/3200000000000 - 16010785891/800000000000000))/(9*((9*3^(1/2))/50000000000000 - 93/200000000000000)) + (100*((3*3^(1/2))/10000 - 11/20000)*((3210399*3^(1/2))/800000000000000 - (3*3^(1/2)*((3*3^(1/2))/20 - 1/10))/2000000000 + 4331121/160000000000000))/(9*((3*3^(1/2))/100000000 - 31/400000000)) + (100*((3*3^(1/2))/2000 + 1/1600)*((5185251*3^(1/2))/16000000000000000 + 31944083711/1600000000000000))/(9*((3*3^(1/2))/100000000 - 31/400000000)) - (100*((3*3^(1/2))/10000 - 11/20000)*((3*3^(1/2))/4000000 - 31/16000000)*((5185251*3^(1/2))/16000000000000000 + 31944083711/1600000000000000))/(9*((3*3^(1/2))/100000000 - 31/400000000)^2) - (20*((27009*3^(1/2))/1000000000 - 3489/50000000)*((99*3^(1/2))/10000000000000 - 1023/40000000000000)*((1183480443*3^(1/2))/80000000000000000 + (21*3^(1/2)*((3*3^(1/2))/20 - 1/10))/3200000000000 - 16010785891/800000000000000))/(9*((9*3^(1/2))/50000000000000 - 93/200000000000000)^2)), 	-T_dis*(((114343521*3^(1/2))/1600000000000000 + (9943777*3^(1/2)*((3*3^(1/2))/20 - 1/10))/20000000000000 + 268316551/800000000000000)/(200*((3*3^(1/2))/100000000 - 31/400000000)) - (20*((27009*3^(1/2))/1000000000 - 3489/50000000)*((2404758213*3^(1/2))/16000000000000000 - (21*3^(1/2)*((3*3^(1/2))/20 - 1/10))/320000000000 + 7131903/64000000000000))/(9*((9*3^(1/2))/50000000000000 - 93/200000000000000)) + (100*((3*3^(1/2))/10000 - 11/20000)*((3465639*3^(1/2))/1600000000000000 + (3*3^(1/2)*((3*3^(1/2))/20 - 1/10))/2000000000 - 55575441/160000000000000))/(9*((3*3^(1/2))/100000000 - 31/400000000)) - (((3*3^(1/2))/5000000 - 31/20000000)*((1665944541*3^(1/2))/32000000000000000 + (3831*3^(1/2)*((3*3^(1/2))/20 - 1/10))/200000000000000 - 160128933757/8000000000000000))/(200*((3*3^(1/2))/100000000 - 31/400000000)^2) + (20*((9*3^(1/2))/25000000 - 213/200000000)*((1183480443*3^(1/2))/80000000000000000 + (21*3^(1/2)*((3*3^(1/2))/20 - 1/10))/3200000000000 - 16010785891/800000000000000))/(9*((9*3^(1/2))/50000000000000 - 93/200000000000000)) + (100*((3*3^(1/2))/500 - 31/2000)*((5185251*3^(1/2))/16000000000000000 + 31944083711/1600000000000000))/(9*((3*3^(1/2))/100000000 - 31/400000000)) - (100*((3*3^(1/2))/10000 - 11/20000)*((3*3^(1/2))/5000000 - 31/20000000)*((5185251*3^(1/2))/16000000000000000 + 31944083711/1600000000000000))/(9*((3*3^(1/2))/100000000 - 31/400000000)^2) - (20*((9*3^(1/2))/1250000000000 - 93/5000000000000)*((27009*3^(1/2))/1000000000 - 3489/50000000)*((1183480443*3^(1/2))/80000000000000000 + (21*3^(1/2)*((3*3^(1/2))/20 - 1/10))/3200000000000 - 16010785891/800000000000000))/(9*((9*3^(1/2))/50000000000000 - 93/200000000000000)^2)), 	T_dis*((20201563*((3*3^(1/2))/10000 - 11/20000))/(960000000*((3*3^(1/2))/100000000 - 31/400000000)) + ((62493*3^(1/2))/16000000000 + (249937*3^(1/2)*((3*3^(1/2))/20 - 1/10))/100000000 - 23974611/32000000000)/(200*((3*3^(1/2))/100000000 - 31/400000000)) - (20*((27009*3^(1/2))/1000000000 - 3489/50000000)*((207*3^(1/2))/1280000000 + (21*3^(1/2)*((3*3^(1/2))/20 - 1/10))/32000000 + 2114643/32000000000))/(9*((9*3^(1/2))/50000000000000 - 93/200000000000000))), 	T_dis*(((3*3^(1/2)*((3*3^(1/2))/20 - 1/10))/8000000000 - (596441019*3^(1/2))/160000000000 + 204842381/80000000000)/(200*((3*3^(1/2))/100000000 - 31/400000000)) + (20*((27009*3^(1/2))/1000000000 - 3489/50000000)*((2107047*3^(1/2))/320000000000 - 168129/12800000000))/(9*((9*3^(1/2))/50000000000000 - 93/200000000000000)) - (100*((3*3^(1/2))/10000 - 11/20000)*((7765251*3^(1/2))/320000000000 + 5703/40000000))/(9*((3*3^(1/2))/100000000 - 31/400000000))), 	-T_dis*(((20010287*3^(1/2)*((3*3^(1/2))/20 - 1/10))/8000000000 - (119986137*3^(1/2))/320000000000 + 40005943/160000000000)/(200*((3*3^(1/2))/100000000 - 31/400000000)) - (100*((416349*3^(1/2))/320000000000 - 123711/32000000000)*((3*3^(1/2))/10000 - 11/20000))/(9*((3*3^(1/2))/100000000 - 31/400000000)) + (20*((27009*3^(1/2))/1000000000 - 3489/50000000)*((1031871*3^(1/2))/1600000000000 - 121359/64000000000))/(9*((9*3^(1/2))/50000000000000 - 93/200000000000000))), 	T_dis*(((7589019*3^(1/2))/500000000000000 + (179409213*3^(1/2)*((3*3^(1/2))/20 - 1/10))/400000000000000 - 125998557/8000000000000000)/(200*((3*3^(1/2))/100000000 - 31/400000000)) + (100*((3*3^(1/2))/10000 - 11/20000)*((4034511*3^(1/2))/1600000000000000 + (297*3^(1/2)*((3*3^(1/2))/20 - 1/10))/400000000000 + 16684749/16000000000000000))/(9*((3*3^(1/2))/100000000 - 31/400000000)) - (20*((27009*3^(1/2))/1000000000 - 3489/50000000)*((52161039*3^(1/2))/3200000000000000 + (21*3^(1/2)*((3*3^(1/2))/20 - 1/10))/32000000000000 - 117174411/8000000000000000))/(9*((9*3^(1/2))/50000000000000 - 93/200000000000000))), 	T_dis*(((1665944541*3^(1/2))/32000000000000000 + (3831*3^(1/2)*((3*3^(1/2))/20 - 1/10))/200000000000000 - 160128933757/8000000000000000)/(300*((3*3^(1/2))/100000000 - 31/400000000)) - ((1183480443*3^(1/2))/80000000000000000 + (21*3^(1/2)*((3*3^(1/2))/20 - 1/10))/3200000000000 - 16010785891/800000000000000)/(50000000*((9*3^(1/2))/50000000000000 - 93/200000000000000)) + ((23697*3^(1/2)*((3*3^(1/2))/20 - 1/10))/32000000000000 - (369986349*3^(1/2))/8000000000000000 + 51614439/8000000000000000)/(200*((3*3^(1/2))/100000000 - 31/400000000)) + (20*((27009*3^(1/2))/1000000000 - 3489/50000000)*((29906877*3^(1/2))/1600000000000000 + (21*3^(1/2)*((3*3^(1/2))/20 - 1/10))/32000000000000 + 5990219349/80000000000000000))/(9*((9*3^(1/2))/50000000000000 - 93/200000000000000)) - (100*((3*3^(1/2))/10000 - 11/20000)*((78898791*3^(1/2))/4000000000000000 + (21*3^(1/2)*((3*3^(1/2))/20 - 1/10))/16000000000000 + 2373464247/20000000000000000))/(9*((3*3^(1/2))/100000000 - 31/400000000))), 	-T_dis*(((599887743*3^(1/2))/16000000000000000 - (1779879*3^(1/2)*((3*3^(1/2))/20 - 1/10))/1600000000000000 + 14540151/32000000000000000)/(200*((3*3^(1/2))/100000000 - 31/400000000)) - (20*((27009*3^(1/2))/1000000000 - 3489/50000000)*((29900577*3^(1/2))/1600000000000000 + (21*3^(1/2)*((3*3^(1/2))/20 - 1/10))/32000000000000 + 5997450849/80000000000000000))/(9*((9*3^(1/2))/50000000000000 - 93/200000000000000)) + (100*((3*3^(1/2))/10000 - 11/20000)*((11901*3^(1/2)*((3*3^(1/2))/20 - 1/10))/32000000000000 - (4750881*3^(1/2))/2000000000000000 + 4731132549/80000000000000000))/(9*((3*3^(1/2))/100000000 - 31/400000000)) + (100*((3*3^(1/2))/20000 - 1/20000)*((1665944541*3^(1/2))/32000000000000000 + (3831*3^(1/2)*((3*3^(1/2))/20 - 1/10))/200000000000000 - 160128933757/8000000000000000))/(3*((3*3^(1/2))/100000000 - 31/400000000)) + (((11*3^(1/2))/200000000 - 3/40000000)*((1665944541*3^(1/2))/32000000000000000 + (3831*3^(1/2)*((3*3^(1/2))/20 - 1/10))/200000000000000 - 160128933757/8000000000000000))/(200*((3*3^(1/2))/100000000 - 31/400000000)^2) - (20*((99*3^(1/2))/2000000 - 27/400000)*((1183480443*3^(1/2))/80000000000000000 + (21*3^(1/2)*((3*3^(1/2))/20 - 1/10))/3200000000000 - 16010785891/800000000000000))/(9*((9*3^(1/2))/50000000000000 - 93/200000000000000)) + (100*((9*3^(1/2))/20000 - 3/20000)*((5185251*3^(1/2))/16000000000000000 + 31944083711/1600000000000000))/(9*((3*3^(1/2))/100000000 - 31/400000000)) + (100*((3*3^(1/2))/10000 - 11/20000)*((11*3^(1/2))/200000000 - 3/40000000)*((5185251*3^(1/2))/16000000000000000 + 31944083711/1600000000000000))/(9*((3*3^(1/2))/100000000 - 31/400000000)^2) + (20*((27009*3^(1/2))/1000000000 - 3489/50000000)*((33*3^(1/2))/100000000000000 - 9/20000000000000)*((1183480443*3^(1/2))/80000000000000000 + (21*3^(1/2)*((3*3^(1/2))/20 - 1/10))/3200000000000 - 16010785891/800000000000000))/(9*((9*3^(1/2))/50000000000000 - 93/200000000000000)^2)), 	T_dis*(((891*3^(1/2))/80000000 - 417/40000000)/(200*((3*3^(1/2))/100000000 - 31/400000000)) - (20*((27009*3^(1/2))/1000000000 - 3489/50000000)*((1192731*3^(1/2))/3200000000 - 1205067/3200000000))/(9*((9*3^(1/2))/50000000000000 - 93/200000000000000)) + (100*((3*3^(1/2))/10000 - 11/20000)*((292941*3^(1/2))/800000000 - 589209/1600000000))/(9*((3*3^(1/2))/100000000 - 31/400000000))), 	T_dis*(((307161*3^(1/2))/800000000 - 620169/1600000000)/(200*((3*3^(1/2))/100000000 - 31/400000000)) - (20*((27009*3^(1/2))/1000000000 - 3489/50000000)*((58929*3^(1/2))/160000000 - 601209/1600000000))/(9*((9*3^(1/2))/50000000000000 - 93/200000000000000)) + (3^(1/2)*((3*3^(1/2))/10000 - 11/20000))/(20000*((3*3^(1/2))/100000000 - 31/400000000))), 	T_dis*(((1192731*3^(1/2))/3200000000 - 1205067/3200000000)/(200*((3*3^(1/2))/100000000 - 31/400000000)) - (100*((3*3^(1/2))/10000 - 11/20000)*((58929*3^(1/2))/160000000 - 601209/1600000000))/(9*((3*3^(1/2))/100000000 - 31/400000000))) + 1, 	0, 	0, 	0, 	0, 	0, 	0, 	0, 	0, 	0, 	0, 	0, 	0, 	T_dis/(200*((3*3^(1/2))/100000000 - 31/400000000)), 	-(100*T_dis*((3*3^(1/2))/10000 - 11/20000))/(9*((3*3^(1/2))/100000000 - 31/400000000)), 	(20*T_dis*((27009*3^(1/2))/1000000000 - 3489/50000000))/(9*((9*3^(1/2))/50000000000000 - 93/200000000000000)), 	T_dis/(200*((3*3^(1/2))/100000000 - 31/400000000)), 	-(100*T_dis*((3*3^(1/2))/10000 - 11/20000))/(9*((3*3^(1/2))/100000000 - 31/400000000)), 	(20*T_dis*((27009*3^(1/2))/1000000000 - 3489/50000000))/(9*((9*3^(1/2))/50000000000000 - 93/200000000000000)); 
		0, 	0, 	0, 	0, 	0, 	0, 	0, 	0, 	0, 	0, 	0, 	0, 	0, 	0, 	0, 	0, 	0, 	0, 	1, 	0, 	0, 	0, 	0, 	0, 	0, 	0, 	0, 	0, 	0, 	0, 	0, 	0, 	0, 	0, 	0, 	0; 
		0, 	0, 	0, 	0, 	0, 	0, 	0, 	0, 	0, 	0, 	0, 	0, 	0, 	0, 	0, 	0, 	0, 	0, 	0, 	1, 	0, 	0, 	0, 	0, 	0, 	0, 	0, 	0, 	0, 	0, 	0, 	0, 	0, 	0, 	0, 	0; 
		0, 	0, 	0, 	0, 	0, 	0, 	0, 	0, 	0, 	0, 	0, 	0, 	0, 	0, 	0, 	0, 	0, 	0, 	0, 	0, 	1, 	0, 	0, 	0, 	0, 	0, 	0, 	0, 	0, 	0, 	0, 	0, 	0, 	0, 	0, 	0; 
		0, 	0, 	0, 	0, 	0, 	0, 	0, 	0, 	0, 	0, 	0, 	0, 	0, 	0, 	0, 	0, 	0, 	0, 	0, 	0, 	0, 	1, 	0, 	0, 	0, 	0, 	0, 	0, 	0, 	0, 	0, 	0, 	0, 	0, 	0, 	0; 
		0, 	0, 	0, 	0, 	0, 	0, 	0, 	0, 	0, 	0, 	0, 	0, 	0, 	0, 	0, 	0, 	0, 	0, 	0, 	0, 	0, 	0, 	1, 	0, 	0, 	0, 	0, 	0, 	0, 	0, 	0, 	0, 	0, 	0, 	0, 	0; 
		0, 	0, 	0, 	0, 	0, 	0, 	0, 	0, 	0, 	0, 	0, 	0, 	0, 	0, 	0, 	0, 	0, 	0, 	0, 	0, 	0, 	0, 	0, 	1, 	0, 	0, 	0, 	0, 	0, 	0, 	0, 	0, 	0, 	0, 	0, 	0; 
		0, 	0, 	0, 	0, 	0, 	0, 	0, 	0, 	0, 	0, 	0, 	0, 	0, 	0, 	0, 	0, 	0, 	0, 	0, 	0, 	0, 	0, 	0, 	0, 	1, 	0, 	0, 	0, 	0, 	0, 	0, 	0, 	0, 	0, 	0, 	0; 
		0, 	0, 	0, 	0, 	0, 	0, 	0, 	0, 	0, 	0, 	0, 	0, 	0, 	0, 	0, 	0, 	0, 	0, 	0, 	0, 	0, 	0, 	0, 	0, 	0, 	1, 	0, 	0, 	0, 	0, 	0, 	0, 	0, 	0, 	0, 	0; 
		0, 	0, 	0, 	0, 	0, 	0, 	0, 	0, 	0, 	0, 	0, 	0, 	0, 	0, 	0, 	0, 	0, 	0, 	0, 	0, 	0, 	0, 	0, 	0, 	0, 	0, 	1, 	0, 	0, 	0, 	0, 	0, 	0, 	0, 	0, 	0; 
		0, 	0, 	0, 	0, 	0, 	0, 	0, 	0, 	0, 	0, 	0, 	0, 	0, 	0, 	0, 	0, 	0, 	0, 	0, 	0, 	0, 	0, 	0, 	0, 	0, 	0, 	0, 	1, 	0, 	0, 	0, 	0, 	0, 	0, 	0, 	0; 
		0, 	0, 	0, 	0, 	0, 	0, 	0, 	0, 	0, 	0, 	0, 	0, 	0, 	0, 	0, 	0, 	0, 	0, 	0, 	0, 	0, 	0, 	0, 	0, 	0, 	0, 	0, 	0, 	1, 	0, 	0, 	0, 	0, 	0, 	0, 	0; 
		0, 	0, 	0, 	0, 	0, 	0, 	0, 	0, 	0, 	0, 	0, 	0, 	0, 	0, 	0, 	0, 	0, 	0, 	0, 	0, 	0, 	0, 	0, 	0, 	0, 	0, 	0, 	0, 	0, 	1, 	0, 	0, 	0, 	0, 	0, 	0; 
		0, 	0, 	0, 	0, 	0, 	0, 	0, 	0, 	0, 	0, 	0, 	0, 	0, 	0, 	0, 	0, 	0, 	0, 	0, 	0, 	0, 	0, 	0, 	0, 	0, 	0, 	0, 	0, 	0, 	0, 	1, 	0, 	0, 	0, 	0, 	0; 
		0, 	0, 	0, 	0, 	0, 	0, 	0, 	0, 	0, 	0, 	0, 	0, 	0, 	0, 	0, 	0, 	0, 	0, 	0, 	0, 	0, 	0, 	0, 	0, 	0, 	0, 	0, 	0, 	0, 	0, 	0, 	1, 	0, 	0, 	0, 	0; 
		0, 	0, 	0, 	0, 	0, 	0, 	0, 	0, 	0, 	0, 	0, 	0, 	0, 	0, 	0, 	0, 	0, 	0, 	0, 	0, 	0, 	0, 	0, 	0, 	0, 	0, 	0, 	0, 	0, 	0, 	0, 	0, 	1, 	0, 	0, 	0; 
		0, 	0, 	0, 	0, 	0, 	0, 	0, 	0, 	0, 	0, 	0, 	0, 	0, 	0, 	0, 	0, 	0, 	0, 	0, 	0, 	0, 	0, 	0, 	0, 	0, 	0, 	0, 	0, 	0, 	0, 	0, 	0, 	0, 	1, 	0, 	0; 
		0, 	0, 	0, 	0, 	0, 	0, 	0, 	0, 	0, 	0, 	0, 	0, 	0, 	0, 	0, 	0, 	0, 	0, 	0, 	0, 	0, 	0, 	0, 	0, 	0, 	0, 	0, 	0, 	0, 	0, 	0, 	0, 	0, 	0, 	1, 	0; 
		0, 	0, 	0, 	0, 	0, 	0, 	0, 	0, 	0, 	0, 	0, 	0, 	0, 	0, 	0, 	0, 	0, 	0, 	0, 	0, 	0, 	0, 	0, 	0, 	0, 	0, 	0, 	0, 	0, 	0, 	0, 	0, 	0, 	0, 	0, 	1];
